simulink model "FO_CTDNN_P_Bia_Para_3_trigger_V1"  (R2021b)
settings: Solver=ode5  StartTime=0.0  StopTime=40  FixedStep=0.005  RelTol=1e-3
(part 1 of 2)
settings Model: Creator=a1752760  LastModifiedBy=a1752760
settings SolverCC: AlgebraicLoopSolver=TrustRegion
settings DebuggingCC: SFMachineParentedDataDiag=warning

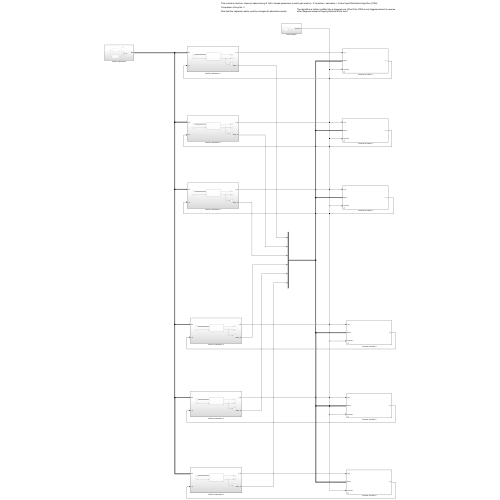
[thumbnail: Simulink's stored preview of the top-level diagram]
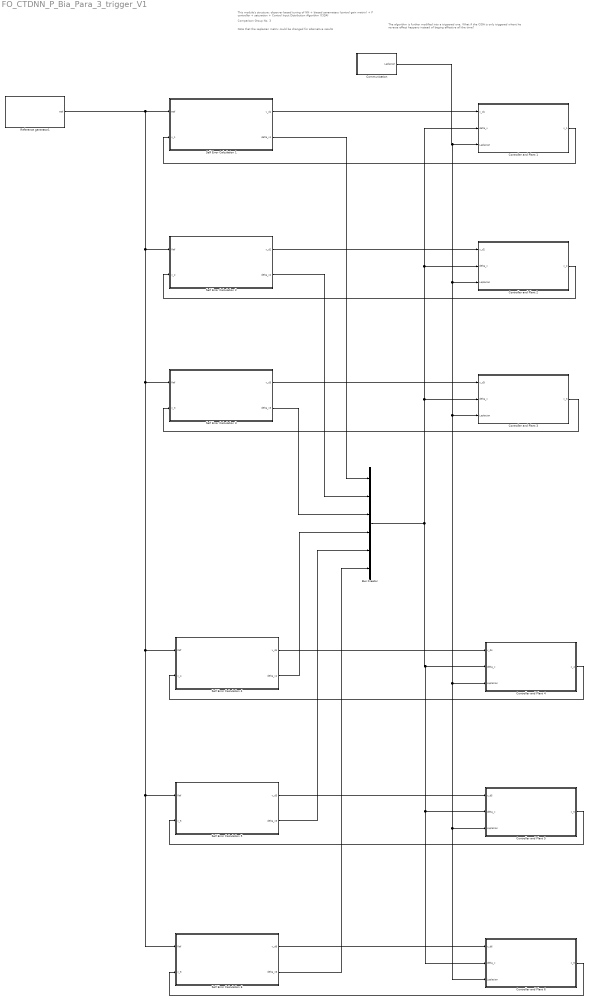
== system FO_CTDNN_P_Bia_Para_3_trigger_V1 ==
  note: The algorithm is further modified into a triggered one. What if the CIDA is only triggered whent he reverse
      | effect happens instead of beging effective all the time?
  note: Comparison Group No. 3
  note: This module's structure: observer based tuning of NN + biased parameters (control gain matrix) + P controller + saturation + Control Input Distribution Algorithm (CIDA)
  note: Note that the Laplacian matrix could be changed for alternative results
  Bus Creator : BusCreator  Inputs=6
  Communication : Subsystem
  Controller and Plant 1 : Subsystem  mask{InitialCondition=[-0.2;-0.7;-pi/4], UpperLimit=0.25, LowerLimit=-0.25}
      mask prompts: InitialCondition "Simulink:blkprm_prompts:IntegratorInitCond"; UpperLimit "Simulink:blkprm_prompts:SaturateUpLim"; LowerLimit "Simulink:blkprm_prompts:SaturateLowLim"
      mask TypeOptions InitialCondition: x_int/InitialCondition
      mask TypeOptions UpperLimit: Saturation/UpperLimit
      mask TypeOptions LowerLimit: Saturation/LowerLimit
      mask DialogControl InitialCondition Prompt: Initial condition:
      mask DialogControl UpperLimit Prompt: Upper limit:
      mask DialogControl LowerLimit Prompt: Lower limit:
  Controller and Plant 2 : Subsystem  mask{InitialCondition=[1.6;3.6;-pi/5], UpperLimit=0.25, LowerLimit=-0.25}
      mask prompts: InitialCondition "Simulink:blkprm_prompts:IntegratorInitCond"; UpperLimit "Simulink:blkprm_prompts:SaturateUpLim"; LowerLimit "Simulink:blkprm_prompts:SaturateLowLim"
      mask TypeOptions InitialCondition: x_int/InitialCondition
      mask TypeOptions UpperLimit: Saturation/UpperLimit
      mask TypeOptions LowerLimit: Saturation/LowerLimit
      mask DialogControl InitialCondition Prompt: Initial condition:
      mask DialogControl UpperLimit Prompt: Upper limit:
      mask DialogControl LowerLimit Prompt: Lower limit:
  Controller and Plant 3 : Subsystem  mask{InitialCondition=[-4;-2.4;pi/3], UpperLimit=0.25, LowerLimit=-0.25}
      mask prompts: InitialCondition "Simulink:blkprm_prompts:IntegratorInitCond"; UpperLimit "Simulink:blkprm_prompts:SaturateUpLim"; LowerLimit "Simulink:blkprm_prompts:SaturateLowLim"
      mask TypeOptions InitialCondition: x_int/InitialCondition
      mask TypeOptions UpperLimit: Saturation/UpperLimit
      mask TypeOptions LowerLimit: Saturation/LowerLimit
      mask DialogControl InitialCondition Prompt: Initial condition:
      mask DialogControl UpperLimit Prompt: Upper limit:
      mask DialogControl LowerLimit Prompt: Lower limit:
  Controller and Plant 4 : Subsystem  mask{InitialCondition=[-1.9;-1.1;pi/4], UpperLimit=0.25, LowerLimit=-0.25}
      mask prompts: InitialCondition "Simulink:blkprm_prompts:IntegratorInitCond"; UpperLimit "Simulink:blkprm_prompts:SaturateUpLim"; LowerLimit "Simulink:blkprm_prompts:SaturateLowLim"
      mask TypeOptions InitialCondition: x_int/InitialCondition
      mask TypeOptions UpperLimit: Saturation/UpperLimit
      mask TypeOptions LowerLimit: Saturation/LowerLimit
      mask DialogControl InitialCondition Prompt: Initial condition:
      mask DialogControl UpperLimit Prompt: Upper limit:
      mask DialogControl LowerLimit Prompt: Lower limit:
  Controller and Plant 5 : Subsystem  mask{InitialCondition=[-1.6;-4.6;-pi/3], UpperLimit=0.25, LowerLimit=-0.25}
      mask prompts: InitialCondition "Simulink:blkprm_prompts:IntegratorInitCond"; UpperLimit "Simulink:blkprm_prompts:SaturateUpLim"; LowerLimit "Simulink:blkprm_prompts:SaturateLowLim"
      mask TypeOptions InitialCondition: x_int/InitialCondition
      mask TypeOptions UpperLimit: Saturation/UpperLimit
      mask TypeOptions LowerLimit: Saturation/LowerLimit
      mask DialogControl InitialCondition Prompt: Initial condition:
      mask DialogControl UpperLimit Prompt: Upper limit:
      mask DialogControl LowerLimit Prompt: Lower limit:
  Controller and Plant 6 : Subsystem  mask{InitialCondition=[3.6;-1.5;-pi/6], UpperLimit=0.25, LowerLimit=-0.25}
      mask prompts: InitialCondition "Simulink:blkprm_prompts:IntegratorInitCond"; UpperLimit "Simulink:blkprm_prompts:SaturateUpLim"; LowerLimit "Simulink:blkprm_prompts:SaturateLowLim"
      mask TypeOptions InitialCondition: x_int/InitialCondition
      mask TypeOptions UpperLimit: Saturation/UpperLimit
      mask TypeOptions LowerLimit: Saturation/LowerLimit
      mask DialogControl InitialCondition Prompt: Initial condition:
      mask DialogControl UpperLimit Prompt: Upper limit:
      mask DialogControl LowerLimit Prompt: Lower limit:
  Reference generator1 : Subsystem
  Self Error Calculation 1 : Subsystem
  Self Error Calculation 2 : Subsystem
  Self Error Calculation 3 : Subsystem
  Self Error Calculation 4 : Subsystem
  Self Error Calculation 5 : Subsystem
  Self Error Calculation 6 : Subsystem
  wires:
  Reference generator1/1(Ref) -> Self Error Calculation 6/1(Ref), Self Error Calculation 5/1(Ref), Self Error Calculation 4/1(Ref), Self Error Calculation 3/1(Ref), Self Error Calculation 2/1(Ref), Self Error Calculation 1/1(Ref)
  Self Error Calculation 1/1(v_d1) -> Controller and Plant 1/1(v_d1)
  Controller and Plant 1/1(x_1) -> Self Error Calculation 1/2(x_1)
  Controller and Plant 2/1(x_2) -> Self Error Calculation 2/2(x_2)
  Self Error Calculation 2/1(v_d2) -> Controller and Plant 2/1(v_d2)
  Controller and Plant 3/1(x_3) -> Self Error Calculation 3/2(x_3)
  Self Error Calculation 3/1(v_d3) -> Controller and Plant 3/1(v_d3)
  Controller and Plant 4/1(x_4) -> Self Error Calculation 4/2(x_4)
  Self Error Calculation 4/1(v_d4) -> Controller and Plant 4/1(v_d4)
  Controller and Plant 5/1(x_5) -> Self Error Calculation 5/2(x_5)
  Self Error Calculation 5/1(v_d5) -> Controller and Plant 5/1(v_d5)
  Controller and Plant 6/1(x_6) -> Self Error Calculation 6/2(x_6)
  Self Error Calculation 6/1(v_d6) -> Controller and Plant 6/1(v_d6)
  Self Error Calculation 1/2(delta_x1) -> Bus Creator/1
  Self Error Calculation 2/2(delta_x2) -> Bus Creator/2
  Self Error Calculation 3/2(delta_x3) -> Bus Creator/3
  Self Error Calculation 4/2(delta_x4) -> Bus Creator/4
  Self Error Calculation 5/2(delta_x5) -> Bus Creator/5
  Self Error Calculation 6/2(delta_x6) -> Bus Creator/6
  Bus Creator/1 -> Controller and Plant 4/2(delta_x), Controller and Plant 6/2(delta_x), Controller and Plant 5/2(delta_x), Controller and Plant 3/2(delta_x), Controller and Plant 2/2(delta_x), Controller and Plant 1/2(delta_x)
  Communication/1(Laplacian) -> Controller and Plant 6/3(Laplacian), Controller and Plant 5/3(Laplacian), Controller and Plant 4/3(Laplacian), Controller and Plant 3/3(Laplacian), Controller and Plant 2/3(Laplacian), Controller and Plant 1/3(Laplacian)

== system FO_CTDNN_P_Bia_Para_3_trigger_V1/Communication ==
  Add : Sum
  Communication Topology : Constant  Value=[2,0,-1,-1,0,0;-1,1,0,0,0,0;0,-1,2,-1,0,0;-1,0,0,3,-1,-1;0,0,0,-1,1,0;-1,0,0,0,0,1]  VectorParams1D=off
  Constant : Constant  Value=2  VectorParams1D=off
  Product : Product
  Reference Feeding : Constant  Value=[1,0,0,0,0,0;0,1,0,0,0,0;0,0,1,0,0,0;0,0,0,1,0,0;0,0,0,0,1,0;0,0,0,0,0,1]  VectorParams1D=off
  Laplacian : Outport  VectorParamsAs1DForOutWhenUnconnected=off
  wires:
  Constant/1 -> Product/2
  Reference Feeding/1 -> Product/1
  Communication Topology/1 -> Add/1
  Product/1 -> Add/2
  Add/1 -> Laplacian/1

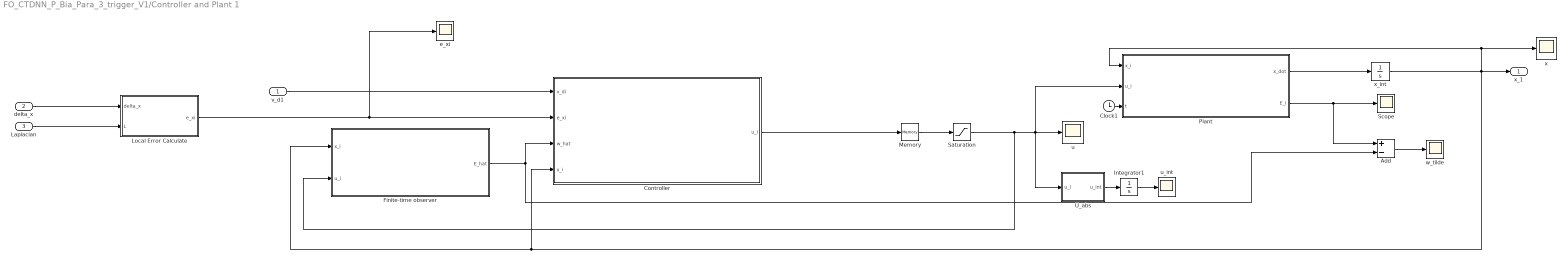
== system FO_CTDNN_P_Bia_Para_3_trigger_V1/Controller and Plant 1 ==
  v_d1 : Inport
  delta_x : Inport  Port=2
  Laplacian : Inport  Port=3
  Add : Sum  Inputs=+-
  Clock1 : Clock
  Controller : Subsystem
  Finite-time observer : Subsystem  mask{InitialCondition=[0;-0.3;-pi/5]}
      mask prompts: InitialCondition "Simulink:blkprm_prompts:IntegratorInitCond"
      mask TypeOptions InitialCondition: Integrator/InitialCondition
      mask DialogControl InitialCondition Prompt: Initial condition:
  Integrator1 : Integrator
  Local Error Calculate : MATLAB Function  TreatAsAtomicUnit=on
  Memory : Memory  InitialCondition=[0;0;0]
  Plant : MATLAB Function  TreatAsAtomicUnit=on
  Saturation : Saturate  UpperLimit=UpperLimit  LowerLimit=LowerLimit
  Scope : Scope
  U_abs : MATLAB Function  TreatAsAtomicUnit=on
  e_xi : Scope
  u : Scope
  u_int : Scope
  w_tilde : Scope
  x : Scope
  x_int : Integrator  InitialCondition=InitialCondition
  x_1 : Outport
  wires:
  Add/1 -> w_tilde/1
  Plant/2(E_i) -> Scope/1, Add/1
  Finite-time observer/1(E_hat) -> Controller/3(w_hat), Add/2
  Clock1/1 -> Plant/3(t)
  Plant/1(x_dot) -> x_int/1
  Memory/1 -> Saturation/1
  x_int/1 -> x_1/1, Plant/1(x_i), x/1, Controller/4(x_i), Finite-time observer/1(x_i)
  v_d1/1 -> Controller/1(v_di)
  Controller/1(u_i) -> Memory/1
  Local Error Calculate/1(e_xi) -> Controller/2(e_xi), e_xi/1
  delta_x/1 -> Local Error Calculate/1(delta_x)
  Laplacian/1 -> Local Error Calculate/2(L)
  Saturation/1 -> Finite-time observer/2(u_i), U_abs/1(u_i), Plant/2(u_i), u/1
  Integrator1/1 -> u_int/1
  U_abs/1(u_int) -> Integrator1/1

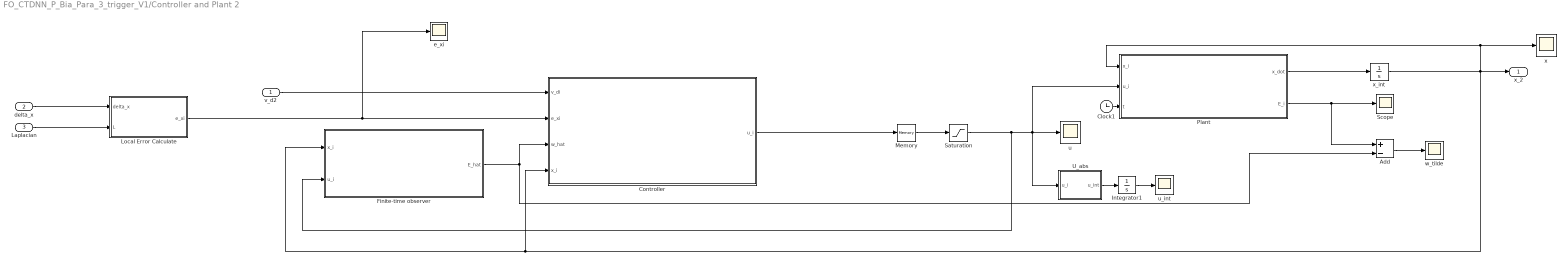
== system FO_CTDNN_P_Bia_Para_3_trigger_V1/Controller and Plant 2 ==
  v_d2 : Inport
  delta_x : Inport  Port=2
  Laplacian : Inport  Port=3
  Add : Sum  Inputs=+-
  Clock1 : Clock
  Controller : Subsystem
  Finite-time observer : Subsystem  mask{InitialCondition=[1.4;3.3;-pi/6]}
      mask prompts: InitialCondition "Simulink:blkprm_prompts:IntegratorInitCond"
      mask TypeOptions InitialCondition: Integrator/InitialCondition
      mask DialogControl InitialCondition Prompt: Initial condition:
  Integrator1 : Integrator
  Local Error Calculate : MATLAB Function  TreatAsAtomicUnit=on
  Memory : Memory  InitialCondition=[0;0;0]
  Plant : MATLAB Function  TreatAsAtomicUnit=on
  Saturation : Saturate  UpperLimit=UpperLimit  LowerLimit=LowerLimit
  Scope : Scope
  U_abs : MATLAB Function  TreatAsAtomicUnit=on
  e_xi : Scope
  u : Scope
  u_int : Scope
  w_tilde : Scope
  x : Scope
  x_int : Integrator  InitialCondition=InitialCondition
  x_2 : Outport
  wires:
  Add/1 -> w_tilde/1
  Plant/2(E_i) -> Scope/1, Add/1
  Finite-time observer/1(E_hat) -> Controller/3(w_hat), Add/2
  Clock1/1 -> Plant/3(t)
  Plant/1(x_dot) -> x_int/1
  Memory/1 -> Saturation/1
  x_int/1 -> x_2/1, Plant/1(x_i), x/1, Controller/4(x_i), Finite-time observer/1(x_i)
  v_d2/1 -> Controller/1(v_di)
  Controller/1(u_i) -> Memory/1
  Local Error Calculate/1(e_xi) -> Controller/2(e_xi), e_xi/1
  delta_x/1 -> Local Error Calculate/1(delta_x)
  Laplacian/1 -> Local Error Calculate/2(L)
  Integrator1/1 -> u_int/1
  Saturation/1 -> Finite-time observer/2(u_i), U_abs/1(u_i), Plant/2(u_i), u/1
  U_abs/1(u_int) -> Integrator1/1

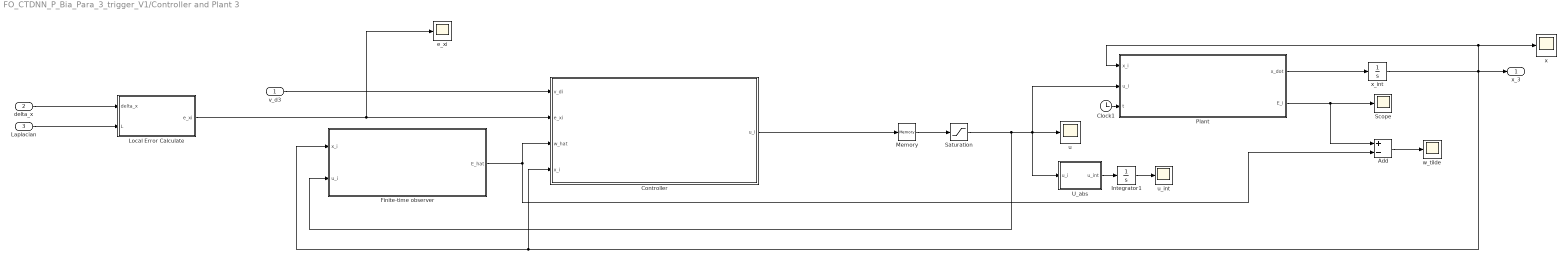
== system FO_CTDNN_P_Bia_Para_3_trigger_V1/Controller and Plant 3 ==
  v_d3 : Inport
  delta_x : Inport  Port=2
  Laplacian : Inport  Port=3
  Add : Sum  Inputs=+-
  Clock1 : Clock
  Controller : Subsystem
  Finite-time observer : Subsystem  mask{InitialCondition=[-3.7;-2.1;pi/4]}
      mask prompts: InitialCondition "Simulink:blkprm_prompts:IntegratorInitCond"
      mask TypeOptions InitialCondition: Integrator/InitialCondition
      mask DialogControl InitialCondition Prompt: Initial condition:
  Integrator1 : Integrator
  Local Error Calculate : MATLAB Function  TreatAsAtomicUnit=on
  Memory : Memory  InitialCondition=[0;0;0]
  Plant : MATLAB Function  TreatAsAtomicUnit=on
  Saturation : Saturate  UpperLimit=UpperLimit  LowerLimit=LowerLimit
  Scope : Scope
  U_abs : MATLAB Function  TreatAsAtomicUnit=on
  e_xi : Scope
  u : Scope
  u_int : Scope
  w_tilde : Scope
  x : Scope
  x_int : Integrator  InitialCondition=InitialCondition
  x_3 : Outport
  wires:
  Add/1 -> w_tilde/1
  Plant/2(E_i) -> Scope/1, Add/1
  Finite-time observer/1(E_hat) -> Controller/3(w_hat), Add/2
  Clock1/1 -> Plant/3(t)
  Plant/1(x_dot) -> x_int/1
  Memory/1 -> Saturation/1
  x_int/1 -> x_3/1, Plant/1(x_i), x/1, Controller/4(x_i), Finite-time observer/1(x_i)
  v_d3/1 -> Controller/1(v_di)
  Controller/1(u_i) -> Memory/1
  Local Error Calculate/1(e_xi) -> Controller/2(e_xi), e_xi/1
  delta_x/1 -> Local Error Calculate/1(delta_x)
  Laplacian/1 -> Local Error Calculate/2(L)
  Integrator1/1 -> u_int/1
  Saturation/1 -> Finite-time observer/2(u_i), U_abs/1(u_i), Plant/2(u_i), u/1
  U_abs/1(u_int) -> Integrator1/1

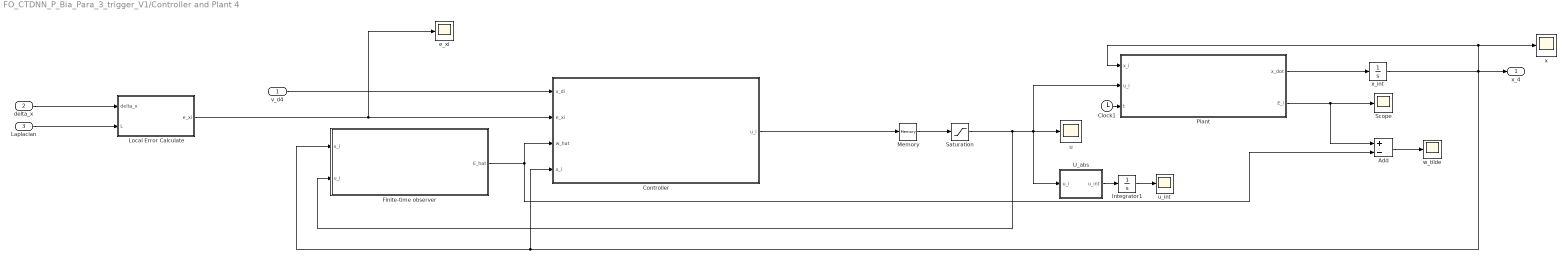
== system FO_CTDNN_P_Bia_Para_3_trigger_V1/Controller and Plant 4 ==
  v_d4 : Inport
  delta_x : Inport  Port=2
  Laplacian : Inport  Port=3
  Add : Sum  Inputs=+-
  Clock1 : Clock
  Controller : Subsystem
  Finite-time observer : Subsystem  mask{InitialCondition=[-1.6;-0.8;pi/6]}
      mask prompts: InitialCondition "Simulink:blkprm_prompts:IntegratorInitCond"
      mask TypeOptions InitialCondition: Integrator/InitialCondition
      mask DialogControl InitialCondition Prompt: Initial condition:
  Integrator1 : Integrator
  Local Error Calculate : MATLAB Function  TreatAsAtomicUnit=on
  Memory : Memory  InitialCondition=[0;0;0]
  Plant : MATLAB Function  TreatAsAtomicUnit=on
  Saturation : Saturate  UpperLimit=UpperLimit  LowerLimit=LowerLimit
  Scope : Scope
  U_abs : MATLAB Function  TreatAsAtomicUnit=on
  e_xi : Scope
  u : Scope
  u_int : Scope
  w_tilde : Scope
  x : Scope
  x_int : Integrator  InitialCondition=InitialCondition
  x_4 : Outport
  wires:
  Add/1 -> w_tilde/1
  Plant/2(E_i) -> Scope/1, Add/1
  Finite-time observer/1(E_hat) -> Controller/3(w_hat), Add/2
  Clock1/1 -> Plant/3(t)
  Plant/1(x_dot) -> x_int/1
  Memory/1 -> Saturation/1
  x_int/1 -> x_4/1, Plant/1(x_i), x/1, Controller/4(x_i), Finite-time observer/1(x_i)
  v_d4/1 -> Controller/1(v_di)
  Controller/1(u_i) -> Memory/1
  Local Error Calculate/1(e_xi) -> Controller/2(e_xi), e_xi/1
  delta_x/1 -> Local Error Calculate/1(delta_x)
  Laplacian/1 -> Local Error Calculate/2(L)
  U_abs/1(u_int) -> Integrator1/1
  Integrator1/1 -> u_int/1
  Saturation/1 -> Finite-time observer/2(u_i), U_abs/1(u_i), Plant/2(u_i), u/1

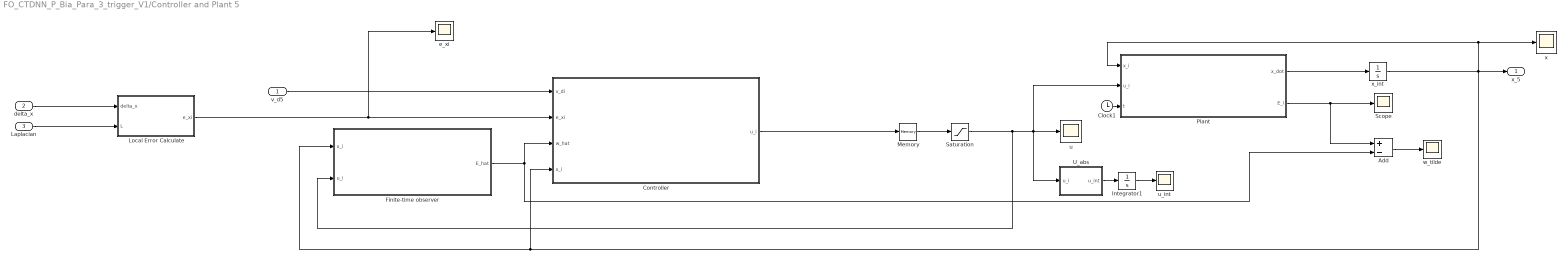
== system FO_CTDNN_P_Bia_Para_3_trigger_V1/Controller and Plant 5 ==
  v_d5 : Inport
  delta_x : Inport  Port=2
  Laplacian : Inport  Port=3
  Add : Sum  Inputs=+-
  Clock1 : Clock
  Controller : Subsystem
  Finite-time observer : Subsystem  mask{InitialCondition=[-1.1;-4.1;-pi/4]}
      mask prompts: InitialCondition "Simulink:blkprm_prompts:IntegratorInitCond"
      mask TypeOptions InitialCondition: Integrator/InitialCondition
      mask DialogControl InitialCondition Prompt: Initial condition:
  Integrator1 : Integrator
  Local Error Calculate : MATLAB Function  TreatAsAtomicUnit=on
  Memory : Memory  InitialCondition=[0;0;0]
  Plant : MATLAB Function  TreatAsAtomicUnit=on
  Saturation : Saturate  UpperLimit=UpperLimit  LowerLimit=LowerLimit
  Scope : Scope
  U_abs : MATLAB Function  TreatAsAtomicUnit=on
  e_xi : Scope
  u : Scope
  u_int : Scope
  w_tilde : Scope
  x : Scope
  x_int : Integrator  InitialCondition=InitialCondition
  x_5 : Outport
  wires:
  Add/1 -> w_tilde/1
  Plant/2(E_i) -> Scope/1, Add/1
  Finite-time observer/1(E_hat) -> Controller/3(w_hat), Add/2
  Clock1/1 -> Plant/3(t)
  Plant/1(x_dot) -> x_int/1
  Memory/1 -> Saturation/1
  x_int/1 -> x_5/1, Plant/1(x_i), x/1, Controller/4(x_i), Finite-time observer/1(x_i)
  v_d5/1 -> Controller/1(v_di)
  Controller/1(u_i) -> Memory/1
  Local Error Calculate/1(e_xi) -> Controller/2(e_xi), e_xi/1
  delta_x/1 -> Local Error Calculate/1(delta_x)
  Laplacian/1 -> Local Error Calculate/2(L)
  U_abs/1(u_int) -> Integrator1/1
  Integrator1/1 -> u_int/1
  Saturation/1 -> Finite-time observer/2(u_i), U_abs/1(u_i), Plant/2(u_i), u/1

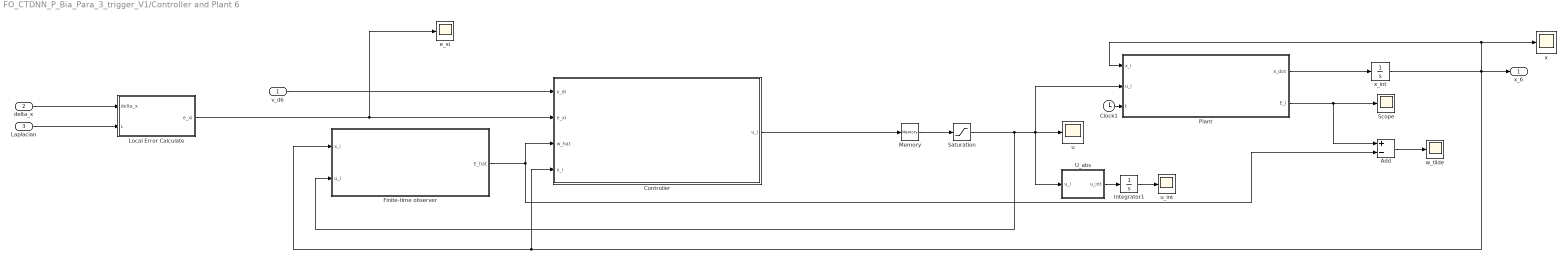
== system FO_CTDNN_P_Bia_Para_3_trigger_V1/Controller and Plant 6 ==
  v_d6 : Inport
  delta_x : Inport  Port=2
  Laplacian : Inport  Port=3
  Add : Sum  Inputs=+-
  Clock1 : Clock
  Controller : Subsystem
  Finite-time observer : Subsystem  mask{InitialCondition=[3.9;-1.9;-pi/5]}
      mask prompts: InitialCondition "Simulink:blkprm_prompts:IntegratorInitCond"
      mask TypeOptions InitialCondition: Integrator/InitialCondition
      mask DialogControl InitialCondition Prompt: Initial condition:
  Integrator1 : Integrator
  Local Error Calculate : MATLAB Function  TreatAsAtomicUnit=on
  Memory : Memory  InitialCondition=[0;0;0]
  Plant : MATLAB Function  TreatAsAtomicUnit=on
  Saturation : Saturate  UpperLimit=UpperLimit  LowerLimit=LowerLimit
  Scope : Scope
  U_abs : MATLAB Function  TreatAsAtomicUnit=on
  e_xi : Scope
  u : Scope
  u_int : Scope
  w_tilde : Scope
  x : Scope
  x_int : Integrator  InitialCondition=InitialCondition
  x_6 : Outport
  wires:
  Add/1 -> w_tilde/1
  Plant/2(E_i) -> Scope/1, Add/1
  Finite-time observer/1(E_hat) -> Controller/3(w_hat), Add/2
  Clock1/1 -> Plant/3(t)
  Plant/1(x_dot) -> x_int/1
  Memory/1 -> Saturation/1
  x_int/1 -> x_6/1, Plant/1(x_i), x/1, Controller/4(x_i), Finite-time observer/1(x_i)
  v_d6/1 -> Controller/1(v_di)
  Controller/1(u_i) -> Memory/1
  Local Error Calculate/1(e_xi) -> Controller/2(e_xi), e_xi/1
  delta_x/1 -> Local Error Calculate/1(delta_x)
  Laplacian/1 -> Local Error Calculate/2(L)
  U_abs/1(u_int) -> Integrator1/1
  Integrator1/1 -> u_int/1
  Saturation/1 -> Finite-time observer/2(u_i), U_abs/1(u_i), Plant/2(u_i), u/1

== system FO_CTDNN_P_Bia_Para_3_trigger_V1/Reference generator1 ==
  Bus Creator : BusCreator  Inputs=2
  Clock : Clock
  Scope : Scope
  reference : MATLAB Function  TreatAsAtomicUnit=on
  reference1 : MATLAB Function  TreatAsAtomicUnit=on
  Ref : Outport
  wires:
  Clock/1 -> reference1/1(t), reference/1(t)
  reference/1(xd) -> Scope/1, Bus Creator/1
  reference1/1(vd) -> Bus Creator/2
  Bus Creator/1 -> Ref/1

== system FO_CTDNN_P_Bia_Para_3_trigger_V1/Self Error Calculation 1 ==
  Ref : Inport
  x_1 : Inport  Port=2
  Scope : Scope
  error_calculation : MATLAB Function  TreatAsAtomicUnit=on
  v_d1 : Outport
  delta_x1 : Outport  Port=2
  wires:
  Ref/1 -> error_calculation/1(ref)
  x_1/1 -> error_calculation/2(x_i)
  error_calculation/1(v_di) -> v_d1/1
  error_calculation/2(delta_x1) -> Scope/1, delta_x1/1

== system FO_CTDNN_P_Bia_Para_3_trigger_V1/Self Error Calculation 2 ==
  Ref : Inport
  x_2 : Inport  Port=2
  Scope : Scope
  error_calculation : MATLAB Function  TreatAsAtomicUnit=on
  v_d2 : Outport
  delta_x2 : Outport  Port=2
  wires:
  Ref/1 -> error_calculation/1(ref)
  x_2/1 -> error_calculation/2(x_i)
  error_calculation/1(v_di) -> v_d2/1
  error_calculation/2(delta_x2) -> Scope/1, delta_x2/1

== system FO_CTDNN_P_Bia_Para_3_trigger_V1/Self Error Calculation 3 ==
  Ref : Inport
  x_3 : Inport  Port=2
  Scope : Scope
  error_calculation : MATLAB Function  TreatAsAtomicUnit=on
  v_d3 : Outport
  delta_x3 : Outport  Port=2
  wires:
  Ref/1 -> error_calculation/1(ref)
  x_3/1 -> error_calculation/2(x_i)
  error_calculation/1(v_di) -> v_d3/1
  error_calculation/2(delta_x3) -> Scope/1, delta_x3/1

== system FO_CTDNN_P_Bia_Para_3_trigger_V1/Self Error Calculation 4 ==
  Ref : Inport
  x_4 : Inport  Port=2
  Scope : Scope
  error_calculation : MATLAB Function  TreatAsAtomicUnit=on
  v_d4 : Outport
  delta_x4 : Outport  Port=2
  wires:
  Ref/1 -> error_calculation/1(ref)
  x_4/1 -> error_calculation/2(x_i)
  error_calculation/1(v_di) -> v_d4/1
  error_calculation/2(delta_x4) -> Scope/1, delta_x4/1

== system FO_CTDNN_P_Bia_Para_3_trigger_V1/Self Error Calculation 5 ==
  Ref : Inport
  x_5 : Inport  Port=2
  Scope : Scope
  error_calculation : MATLAB Function  TreatAsAtomicUnit=on
  v_d5 : Outport
  delta_x5 : Outport  Port=2
  wires:
  Ref/1 -> error_calculation/1(ref)
  x_5/1 -> error_calculation/2(x_i)
  error_calculation/1(v_di) -> v_d5/1
  error_calculation/2(delta_x5) -> Scope/1, delta_x5/1

== system FO_CTDNN_P_Bia_Para_3_trigger_V1/Self Error Calculation 6 ==
  Ref : Inport
  x_6 : Inport  Port=2
  Scope : Scope
  error_calculation : MATLAB Function  TreatAsAtomicUnit=on
  v_d6 : Outport
  delta_x6 : Outport  Port=2
  wires:
  Ref/1 -> error_calculation/1(ref)
  x_6/1 -> error_calculation/2(x_i)
  error_calculation/1(v_di) -> v_d6/1
  error_calculation/2(delta_x6) -> Scope/1, delta_x6/1

== system FO_CTDNN_P_Bia_Para_3_trigger_V1/Controller and Plant 1/Controller ==
  v_di : Inport
  e_xi : Inport  Port=2
  w_hat : Inport  Port=3
  x_i : Inport  Port=4
  Add : Sum
  Control gain matrix : MATLAB Function  TreatAsAtomicUnit=on
  Scope{,1..3} (4 alike) : Scope
  Smooth Projection : MATLAB Function  TreatAsAtomicUnit=on
  controller : MATLAB Function  TreatAsAtomicUnit=on
  u_d,i : MATLAB Function  TreatAsAtomicUnit=on
  u_e,i : MATLAB Function  TreatAsAtomicUnit=on
  u_t,i : MATLAB Function  TreatAsAtomicUnit=on
  xi_i : Scope
  u_i : Outport
  wires:
  x_i/1 -> Control gain matrix/1(x_i)
  Control gain matrix/2(g_inverse) -> u_e,i/1(g_inverse), u_d,i/1(g_inverse), u_t,i/1(g_inverse)
  v_di/1 -> u_t,i/2(v_di)
  w_hat/1 -> Scope3/1, u_d,i/2(w_hat)
  e_xi/1 -> u_e,i/2(e_xi)
  u_e,i/1(u_ei) -> controller/3(u_ei), Scope/1
  controller/1(u_i) -> u_i/1
  controller/2(xi_min) -> xi_i/1
  u_t,i/1(u_ti) -> Add/1
  u_d,i/1(u_di) -> Add/2
  Add/1 -> Scope1/1, Smooth Projection/1("u_mi ")
  Smooth Projection/1(u_mi) -> controller/2(u_mi), Scope2/1
  Control gain matrix/1(g_i_hat) -> controller/1(g_i_hat)

== system FO_CTDNN_P_Bia_Para_3_trigger_V1/Controller and Plant 1/Finite-time observer ==
  x_i : Inport
  u_i : Inport  Port=2
  Integrator : Integrator  InitialCondition=InitialCondition
  Multi-layer neural network : Subsystem
  Observer : MATLAB Function  TreatAsAtomicUnit=on
  x_i_tilde : Scope
  E_hat : Outport
  wires:
  x_i/1 -> Observer/2(x_i), Multi-layer neural network/2(x_i)
  u_i/1 -> Observer/3(u_i), Multi-layer neural network/3(u_i)
  Multi-layer neural network/1(E_hat) -> E_hat/1, Observer/4(E_hat)
  Observer/1(x_hat_dot) -> Integrator/1
  Integrator/1 -> Observer/1(x_i_hat)
  Observer/2(x_i_tilde) -> x_i_tilde/1, Multi-layer neural network/1(x_i_tilde)

== system FO_CTDNN_P_Bia_Para_3_trigger_V1/Controller and Plant 2/Controller ==
  v_di : Inport
  e_xi : Inport  Port=2
  w_hat : Inport  Port=3
  x_i : Inport  Port=4
  Add : Sum
  Control gain matrix : MATLAB Function  TreatAsAtomicUnit=on
  Scope{,1..3} (4 alike) : Scope
  Smooth Projection : MATLAB Function  TreatAsAtomicUnit=on
  controller : MATLAB Function  TreatAsAtomicUnit=on
  u_d,i : MATLAB Function  TreatAsAtomicUnit=on
  u_e,i : MATLAB Function  TreatAsAtomicUnit=on
  u_t,i : MATLAB Function  TreatAsAtomicUnit=on
  xi_i : Scope
  u_i : Outport
  wires:
  x_i/1 -> Control gain matrix/1(x_i)
  Control gain matrix/2(g_inverse) -> u_e,i/1(g_inverse), u_d,i/1(g_inverse), u_t,i/1(g_inverse)
  v_di/1 -> u_t,i/2(v_di)
  w_hat/1 -> Scope3/1, u_d,i/2(w_hat)
  e_xi/1 -> u_e,i/2(e_xi)
  u_e,i/1(u_ei) -> controller/3(u_ei), Scope/1
  controller/1(u_i) -> u_i/1
  controller/2(xi_min) -> xi_i/1
  u_t,i/1(u_ti) -> Add/1
  u_d,i/1(u_di) -> Add/2
  Add/1 -> Scope1/1, Smooth Projection/1("u_mi ")
  Smooth Projection/1(u_mi) -> controller/2(u_mi), Scope2/1
  Control gain matrix/1(g_i_hat) -> controller/1(g_i_hat)

== system FO_CTDNN_P_Bia_Para_3_trigger_V1/Controller and Plant 2/Finite-time observer ==
  x_i : Inport
  u_i : Inport  Port=2
  Integrator : Integrator  InitialCondition=InitialCondition
  Multi-layer neural network : Subsystem
  Observer : MATLAB Function  TreatAsAtomicUnit=on
  x_i_tilde : Scope
  E_hat : Outport
  wires:
  x_i/1 -> Observer/2(x_i), Multi-layer neural network/2(x_i)
  u_i/1 -> Observer/3(u_i), Multi-layer neural network/3(u_i)
  Multi-layer neural network/1(E_hat) -> E_hat/1, Observer/4(E_hat)
  Observer/1(x_hat_dot) -> Integrator/1
  Integrator/1 -> Observer/1(x_i_hat)
  Observer/2(x_i_tilde) -> x_i_tilde/1, Multi-layer neural network/1(x_i_tilde)

== system FO_CTDNN_P_Bia_Para_3_trigger_V1/Controller and Plant 3/Controller ==
  v_di : Inport
  e_xi : Inport  Port=2
  w_hat : Inport  Port=3
  x_i : Inport  Port=4
  Add : Sum
  Control gain matrix : MATLAB Function  TreatAsAtomicUnit=on
  Scope{,1..3} (4 alike) : Scope
  Smooth Projection : MATLAB Function  TreatAsAtomicUnit=on
  controller : MATLAB Function  TreatAsAtomicUnit=on
  u_d,i : MATLAB Function  TreatAsAtomicUnit=on
  u_e,i : MATLAB Function  TreatAsAtomicUnit=on
  u_t,i : MATLAB Function  TreatAsAtomicUnit=on
  xi_i : Scope
  u_i : Outport
  wires:
  x_i/1 -> Control gain matrix/1(x_i)
  Control gain matrix/2(g_inverse) -> u_e,i/1(g_inverse), u_d,i/1(g_inverse), u_t,i/1(g_inverse)
  v_di/1 -> u_t,i/2(v_di)
  w_hat/1 -> Scope3/1, u_d,i/2(w_hat)
  e_xi/1 -> u_e,i/2(e_xi)
  u_e,i/1(u_ei) -> controller/3(u_ei), Scope/1
  controller/1(u_i) -> u_i/1
  controller/2(xi_min) -> xi_i/1
  u_t,i/1(u_ti) -> Add/1
  u_d,i/1(u_di) -> Add/2
  Add/1 -> Scope1/1, Smooth Projection/1("u_mi ")
  Smooth Projection/1(u_mi) -> controller/2(u_mi), Scope2/1
  Control gain matrix/1(g_i_hat) -> controller/1(g_i_hat)

== system FO_CTDNN_P_Bia_Para_3_trigger_V1/Controller and Plant 3/Finite-time observer ==
  x_i : Inport
  u_i : Inport  Port=2
  Integrator : Integrator  InitialCondition=InitialCondition
  Multi-layer neural network : Subsystem
  Observer : MATLAB Function  TreatAsAtomicUnit=on
  x_i_tilde : Scope
  E_hat : Outport
  wires:
  x_i/1 -> Observer/2(x_i), Multi-layer neural network/2(x_i)
  u_i/1 -> Observer/3(u_i), Multi-layer neural network/3(u_i)
  Multi-layer neural network/1(E_hat) -> E_hat/1, Observer/4(E_hat)
  Observer/1(x_hat_dot) -> Integrator/1
  Integrator/1 -> Observer/1(x_i_hat)
  Observer/2(x_i_tilde) -> x_i_tilde/1, Multi-layer neural network/1(x_i_tilde)

== system FO_CTDNN_P_Bia_Para_3_trigger_V1/Controller and Plant 4/Controller ==
  v_di : Inport
  e_xi : Inport  Port=2
  w_hat : Inport  Port=3
  x_i : Inport  Port=4
  Add : Sum
  Control gain matrix : MATLAB Function  TreatAsAtomicUnit=on
  Scope{,1..3} (4 alike) : Scope
  Smooth Projection : MATLAB Function  TreatAsAtomicUnit=on
  controller : MATLAB Function  TreatAsAtomicUnit=on
  u_d,i : MATLAB Function  TreatAsAtomicUnit=on
  u_e,i : MATLAB Function  TreatAsAtomicUnit=on
  u_t,i : MATLAB Function  TreatAsAtomicUnit=on
  xi_i : Scope
  u_i : Outport
  wires:
  x_i/1 -> Control gain matrix/1(x_i)
  Control gain matrix/2(g_inverse) -> u_e,i/1(g_inverse), u_d,i/1(g_inverse), u_t,i/1(g_inverse)
  v_di/1 -> u_t,i/2(v_di)
  w_hat/1 -> Scope3/1, u_d,i/2(w_hat)
  e_xi/1 -> u_e,i/2(e_xi)
  u_e,i/1(u_ei) -> controller/3(u_ei), Scope/1
  controller/1(u_i) -> u_i/1
  controller/2(xi_min) -> xi_i/1
  u_t,i/1(u_ti) -> Add/1
  u_d,i/1(u_di) -> Add/2
  Add/1 -> Scope1/1, Smooth Projection/1("u_mi ")
  Smooth Projection/1(u_mi) -> controller/2(u_mi), Scope2/1
  Control gain matrix/1(g_i_hat) -> controller/1(g_i_hat)

== system FO_CTDNN_P_Bia_Para_3_trigger_V1/Controller and Plant 4/Finite-time observer ==
  x_i : Inport
  u_i : Inport  Port=2
  Integrator : Integrator  InitialCondition=InitialCondition
  Multi-layer neural network : Subsystem
  Observer : MATLAB Function  TreatAsAtomicUnit=on
  x_i_tilde : Scope
  E_hat : Outport
  wires:
  x_i/1 -> Observer/2(x_i), Multi-layer neural network/2(x_i)
  u_i/1 -> Observer/3(u_i), Multi-layer neural network/3(u_i)
  Multi-layer neural network/1(E_hat) -> E_hat/1, Observer/4(E_hat)
  Observer/1(x_hat_dot) -> Integrator/1
  Integrator/1 -> Observer/1(x_i_hat)
  Observer/2(x_i_tilde) -> x_i_tilde/1, Multi-layer neural network/1(x_i_tilde)

== system FO_CTDNN_P_Bia_Para_3_trigger_V1/Controller and Plant 5/Controller ==
  v_di : Inport
  e_xi : Inport  Port=2
  w_hat : Inport  Port=3
  x_i : Inport  Port=4
  Add : Sum
  Control gain matrix : MATLAB Function  TreatAsAtomicUnit=on
  Scope{,1..3} (4 alike) : Scope
  Smooth Projection : MATLAB Function  TreatAsAtomicUnit=on
  controller : MATLAB Function  TreatAsAtomicUnit=on
  u_d,i : MATLAB Function  TreatAsAtomicUnit=on
  u_e,i : MATLAB Function  TreatAsAtomicUnit=on
  u_t,i : MATLAB Function  TreatAsAtomicUnit=on
  xi_i : Scope
  u_i : Outport
  wires:
  x_i/1 -> Control gain matrix/1(x_i)
  Control gain matrix/2(g_inverse) -> u_e,i/1(g_inverse), u_d,i/1(g_inverse), u_t,i/1(g_inverse)
  v_di/1 -> u_t,i/2(v_di)
  w_hat/1 -> Scope3/1, u_d,i/2(w_hat)
  e_xi/1 -> u_e,i/2(e_xi)
  u_e,i/1(u_ei) -> controller/3(u_ei), Scope/1
  controller/1(u_i) -> u_i/1
  controller/2(xi_min) -> xi_i/1
  u_t,i/1(u_ti) -> Add/1
  u_d,i/1(u_di) -> Add/2
  Add/1 -> Scope1/1, Smooth Projection/1("u_mi ")
  Smooth Projection/1(u_mi) -> controller/2(u_mi), Scope2/1
  Control gain matrix/1(g_i_hat) -> controller/1(g_i_hat)

== system FO_CTDNN_P_Bia_Para_3_trigger_V1/Controller and Plant 5/Finite-time observer ==
  x_i : Inport
  u_i : Inport  Port=2
  Integrator : Integrator  InitialCondition=InitialCondition
  Multi-layer neural network : Subsystem
  Observer : MATLAB Function  TreatAsAtomicUnit=on
  x_i_tilde : Scope
  E_hat : Outport
  wires:
  x_i/1 -> Observer/2(x_i), Multi-layer neural network/2(x_i)
  u_i/1 -> Observer/3(u_i), Multi-layer neural network/3(u_i)
  Multi-layer neural network/1(E_hat) -> E_hat/1, Observer/4(E_hat)
  Observer/1(x_hat_dot) -> Integrator/1
  Integrator/1 -> Observer/1(x_i_hat)
  Observer/2(x_i_tilde) -> x_i_tilde/1, Multi-layer neural network/1(x_i_tilde)

== system FO_CTDNN_P_Bia_Para_3_trigger_V1/Controller and Plant 6/Controller ==
  v_di : Inport
  e_xi : Inport  Port=2
  w_hat : Inport  Port=3
  x_i : Inport  Port=4
  Add : Sum
  Control gain matrix : MATLAB Function  TreatAsAtomicUnit=on
  Scope{,1..3} (4 alike) : Scope
  Smooth Projection : MATLAB Function  TreatAsAtomicUnit=on
  controller : MATLAB Function  TreatAsAtomicUnit=on
  u_d,i : MATLAB Function  TreatAsAtomicUnit=on
  u_e,i : MATLAB Function  TreatAsAtomicUnit=on
  u_t,i : MATLAB Function  TreatAsAtomicUnit=on
  xi_i : Scope
  u_i : Outport
  wires:
  x_i/1 -> Control gain matrix/1(x_i)
  Control gain matrix/2(g_inverse) -> u_e,i/1(g_inverse), u_d,i/1(g_inverse), u_t,i/1(g_inverse)
  v_di/1 -> u_t,i/2(v_di)
  w_hat/1 -> Scope3/1, u_d,i/2(w_hat)
  e_xi/1 -> u_e,i/2(e_xi)
  u_e,i/1(u_ei) -> controller/3(u_ei), Scope/1
  controller/1(u_i) -> u_i/1
  controller/2(xi_min) -> xi_i/1
  u_t,i/1(u_ti) -> Add/1
  u_d,i/1(u_di) -> Add/2
  Add/1 -> Scope1/1, Smooth Projection/1("u_mi ")
  Smooth Projection/1(u_mi) -> controller/2(u_mi), Scope2/1
  Control gain matrix/1(g_i_hat) -> controller/1(g_i_hat)

== system FO_CTDNN_P_Bia_Para_3_trigger_V1/Controller and Plant 6/Finite-time observer ==
  x_i : Inport
  u_i : Inport  Port=2
  Integrator : Integrator  InitialCondition=InitialCondition
  Multi-layer neural network : Subsystem
  Observer : MATLAB Function  TreatAsAtomicUnit=on
  x_i_tilde : Scope
  E_hat : Outport
  wires:
  x_i/1 -> Observer/2(x_i), Multi-layer neural network/2(x_i)
  u_i/1 -> Observer/3(u_i), Multi-layer neural network/3(u_i)
  Multi-layer neural network/1(E_hat) -> E_hat/1, Observer/4(E_hat)
  Observer/1(x_hat_dot) -> Integrator/1
  Integrator/1 -> Observer/1(x_i_hat)
  Observer/2(x_i_tilde) -> x_i_tilde/1, Multi-layer neural network/1(x_i_tilde)

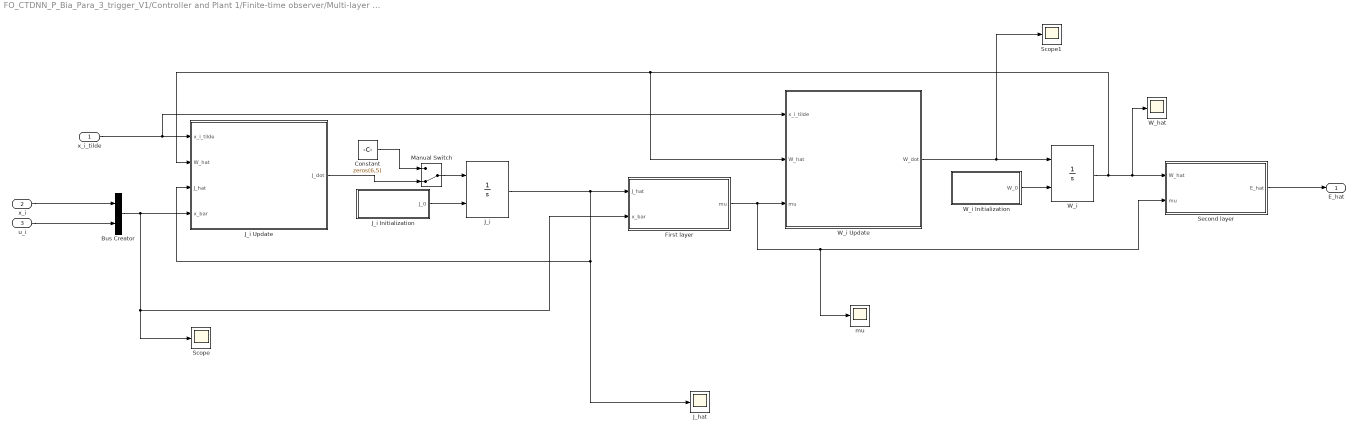
== system FO_CTDNN_P_Bia_Para_3_trigger_V1/Controller and Plant 1/Finite-time observer/Multi-layer neural network ==
  x_i_tilde : Inport
  x_i : Inport  Port=2  PortDimensions=[3,1]
  u_i : Inport  Port=3  PortDimensions=[3,1]
  Bus Creator : BusCreator  Inputs=2
  Constant : Constant  Value=zeros(6,5)
  First layer : MATLAB Function  TreatAsAtomicUnit=on
  J_hat : Scope
  J_i : Integrator  InitialConditionSource=external
  J_i Initialization : MATLAB Function  TreatAsAtomicUnit=on
  J_i Update : MATLAB Function  TreatAsAtomicUnit=on
  Manual Switch : ManualSwitch  CurrentSetting=0
  Scope : Scope
  Scope1 : Scope
  Second layer : MATLAB Function  TreatAsAtomicUnit=on
  W_hat : Scope
  W_i : Integrator  InitialConditionSource=external
  W_i Initialization : MATLAB Function  TreatAsAtomicUnit=on
  W_i Update : MATLAB Function  TreatAsAtomicUnit=on
  mu : Scope
  E_hat : Outport
  wires:
  x_i_tilde/1 -> W_i Update/1(x_i_tilde), J_i Update/1(x_i_tilde)
  W_i/1 -> W_hat/1, Second layer/1(W_hat), W_i Update/2(W_hat), J_i Update/2(W_hat)
  W_i Update/1(W_dot) -> Scope1/1, W_i/1
  W_i Initialization/1(W_0) -> W_i/2
  J_i Initialization/1(J_0) -> J_i/2
  First layer/1(mu) -> mu/1, Second layer/2(mu), W_i Update/3(mu)
  Second layer/1(E_hat) -> E_hat/1
  J_i/1 -> J_i Update/3(J_hat), J_hat/1, First layer/1(J_hat)
  Bus Creator/1 -> Scope/1, First layer/2(x_bar), J_i Update/4(x_bar)
  x_i/1 -> Bus Creator/1
  u_i/1 -> Bus Creator/2
  J_i Update/1(J_dot) -> Manual Switch/2
  Constant/1 -> Manual Switch/1
  Manual Switch/1 -> J_i/1

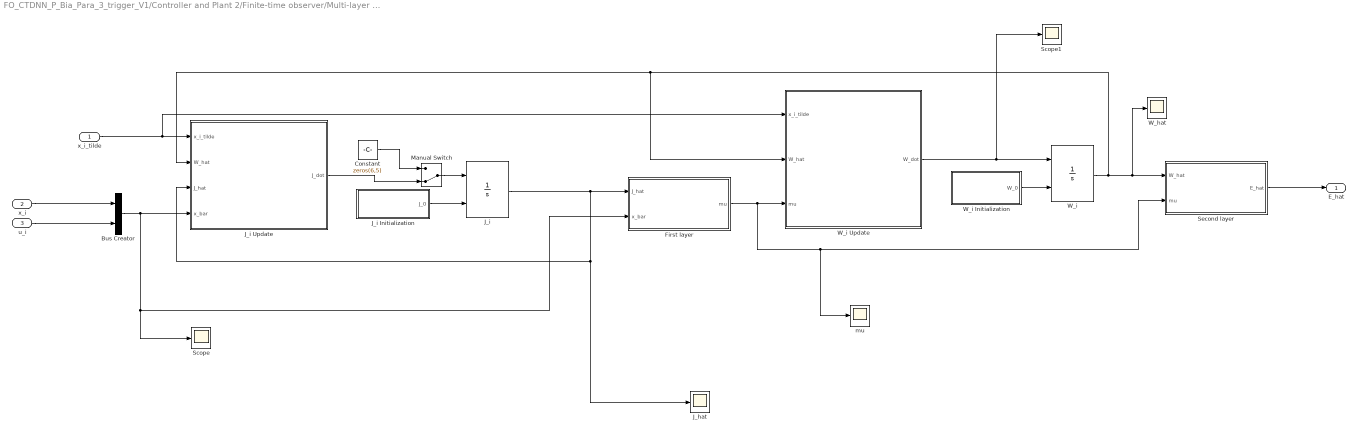
== system FO_CTDNN_P_Bia_Para_3_trigger_V1/Controller and Plant 2/Finite-time observer/Multi-layer neural network ==
  x_i_tilde : Inport
  x_i : Inport  Port=2  PortDimensions=[3,1]
  u_i : Inport  Port=3  PortDimensions=[3,1]
  Bus Creator : BusCreator  Inputs=2
  Constant : Constant  Value=zeros(6,5)
  First layer : MATLAB Function  TreatAsAtomicUnit=on
  J_hat : Scope
  J_i : Integrator  InitialConditionSource=external
  J_i Initialization : MATLAB Function  TreatAsAtomicUnit=on
  J_i Update : MATLAB Function  TreatAsAtomicUnit=on
  Manual Switch : ManualSwitch  CurrentSetting=0
  Scope : Scope
  Scope1 : Scope
  Second layer : MATLAB Function  TreatAsAtomicUnit=on
  W_hat : Scope
  W_i : Integrator  InitialConditionSource=external
  W_i Initialization : MATLAB Function  TreatAsAtomicUnit=on
  W_i Update : MATLAB Function  TreatAsAtomicUnit=on
  mu : Scope
  E_hat : Outport
  wires:
  x_i_tilde/1 -> W_i Update/1(x_i_tilde), J_i Update/1(x_i_tilde)
  W_i/1 -> W_hat/1, Second layer/1(W_hat), W_i Update/2(W_hat), J_i Update/2(W_hat)
  W_i Update/1(W_dot) -> Scope1/1, W_i/1
  W_i Initialization/1(W_0) -> W_i/2
  J_i Initialization/1(J_0) -> J_i/2
  First layer/1(mu) -> mu/1, Second layer/2(mu), W_i Update/3(mu)
  Second layer/1(E_hat) -> E_hat/1
  J_i/1 -> J_i Update/3(J_hat), J_hat/1, First layer/1(J_hat)
  Bus Creator/1 -> Scope/1, First layer/2(x_bar), J_i Update/4(x_bar)
  x_i/1 -> Bus Creator/1
  u_i/1 -> Bus Creator/2
  J_i Update/1(J_dot) -> Manual Switch/2
  Constant/1 -> Manual Switch/1
  Manual Switch/1 -> J_i/1

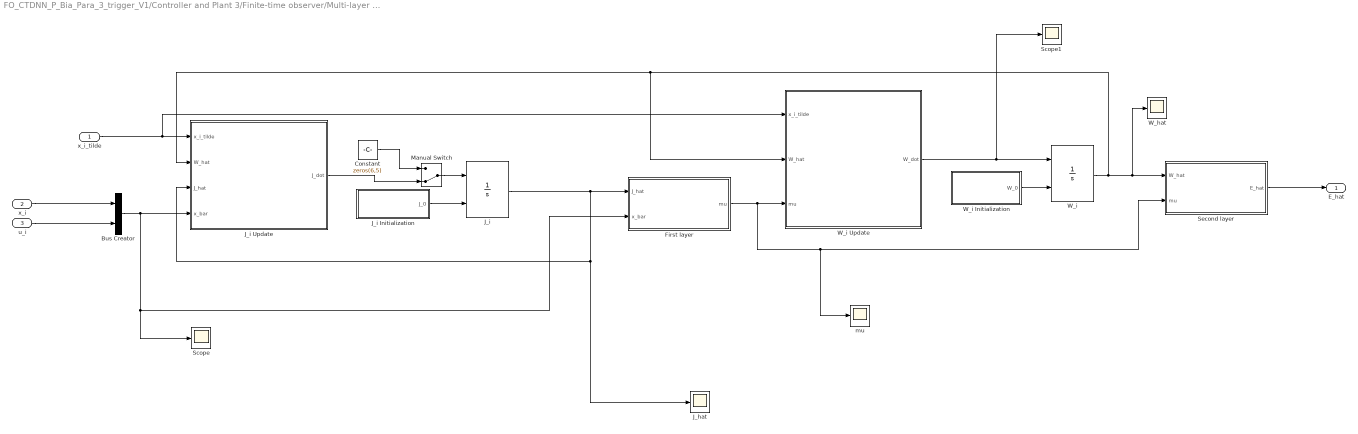
== system FO_CTDNN_P_Bia_Para_3_trigger_V1/Controller and Plant 3/Finite-time observer/Multi-layer neural network ==
  x_i_tilde : Inport
  x_i : Inport  Port=2  PortDimensions=[3,1]
  u_i : Inport  Port=3  PortDimensions=[3,1]
  Bus Creator : BusCreator  Inputs=2
  Constant : Constant  Value=zeros(6,5)
  First layer : MATLAB Function  TreatAsAtomicUnit=on
  J_hat : Scope
  J_i : Integrator  InitialConditionSource=external
  J_i Initialization : MATLAB Function  TreatAsAtomicUnit=on
  J_i Update : MATLAB Function  TreatAsAtomicUnit=on
  Manual Switch : ManualSwitch  CurrentSetting=0
  Scope : Scope
  Scope1 : Scope
  Second layer : MATLAB Function  TreatAsAtomicUnit=on
  W_hat : Scope
  W_i : Integrator  InitialConditionSource=external
  W_i Initialization : MATLAB Function  TreatAsAtomicUnit=on
  W_i Update : MATLAB Function  TreatAsAtomicUnit=on
  mu : Scope
  E_hat : Outport
  wires:
  x_i_tilde/1 -> W_i Update/1(x_i_tilde), J_i Update/1(x_i_tilde)
  W_i/1 -> W_hat/1, Second layer/1(W_hat), W_i Update/2(W_hat), J_i Update/2(W_hat)
  W_i Update/1(W_dot) -> Scope1/1, W_i/1
  W_i Initialization/1(W_0) -> W_i/2
  J_i Initialization/1(J_0) -> J_i/2
  First layer/1(mu) -> mu/1, Second layer/2(mu), W_i Update/3(mu)
  Second layer/1(E_hat) -> E_hat/1
  J_i/1 -> J_i Update/3(J_hat), J_hat/1, First layer/1(J_hat)
  Bus Creator/1 -> Scope/1, First layer/2(x_bar), J_i Update/4(x_bar)
  x_i/1 -> Bus Creator/1
  u_i/1 -> Bus Creator/2
  J_i Update/1(J_dot) -> Manual Switch/2
  Constant/1 -> Manual Switch/1
  Manual Switch/1 -> J_i/1

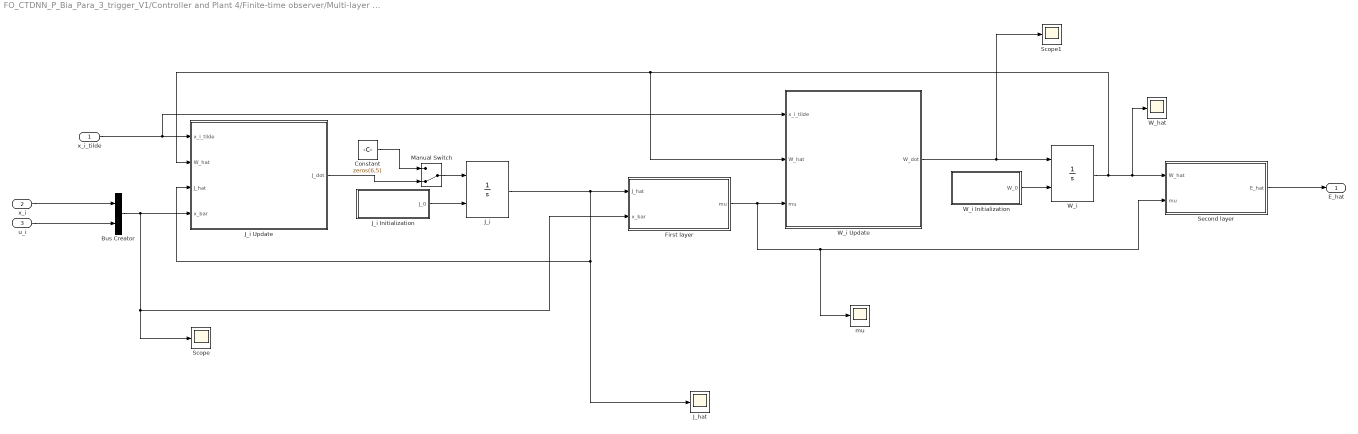
== system FO_CTDNN_P_Bia_Para_3_trigger_V1/Controller and Plant 4/Finite-time observer/Multi-layer neural network ==
  x_i_tilde : Inport
  x_i : Inport  Port=2  PortDimensions=[3,1]
  u_i : Inport  Port=3  PortDimensions=[3,1]
  Bus Creator : BusCreator  Inputs=2
  Constant : Constant  Value=zeros(6,5)
  First layer : MATLAB Function  TreatAsAtomicUnit=on
  J_hat : Scope
  J_i : Integrator  InitialConditionSource=external
  J_i Initialization : MATLAB Function  TreatAsAtomicUnit=on
  J_i Update : MATLAB Function  TreatAsAtomicUnit=on
  Manual Switch : ManualSwitch  CurrentSetting=0
  Scope : Scope
  Scope1 : Scope
  Second layer : MATLAB Function  TreatAsAtomicUnit=on
  W_hat : Scope
  W_i : Integrator  InitialConditionSource=external
  W_i Initialization : MATLAB Function  TreatAsAtomicUnit=on
  W_i Update : MATLAB Function  TreatAsAtomicUnit=on
  mu : Scope
  E_hat : Outport
  wires:
  x_i_tilde/1 -> W_i Update/1(x_i_tilde), J_i Update/1(x_i_tilde)
  W_i/1 -> W_hat/1, Second layer/1(W_hat), W_i Update/2(W_hat), J_i Update/2(W_hat)
  W_i Update/1(W_dot) -> Scope1/1, W_i/1
  W_i Initialization/1(W_0) -> W_i/2
  J_i Initialization/1(J_0) -> J_i/2
  First layer/1(mu) -> mu/1, Second layer/2(mu), W_i Update/3(mu)
  Second layer/1(E_hat) -> E_hat/1
  J_i/1 -> J_i Update/3(J_hat), J_hat/1, First layer/1(J_hat)
  Bus Creator/1 -> Scope/1, First layer/2(x_bar), J_i Update/4(x_bar)
  x_i/1 -> Bus Creator/1
  u_i/1 -> Bus Creator/2
  J_i Update/1(J_dot) -> Manual Switch/2
  Constant/1 -> Manual Switch/1
  Manual Switch/1 -> J_i/1

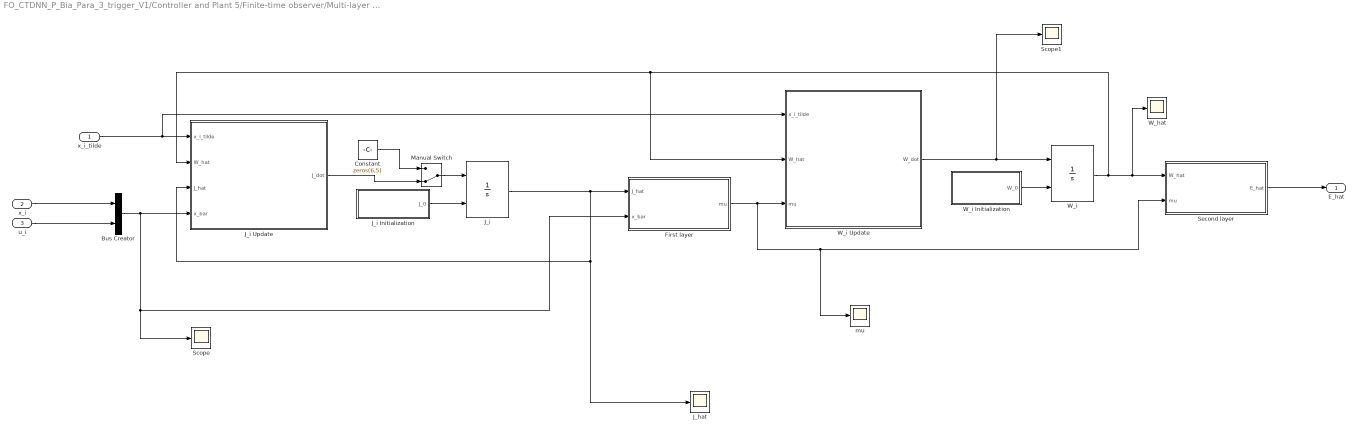
== system FO_CTDNN_P_Bia_Para_3_trigger_V1/Controller and Plant 5/Finite-time observer/Multi-layer neural network ==
  x_i_tilde : Inport
  x_i : Inport  Port=2  PortDimensions=[3,1]
  u_i : Inport  Port=3  PortDimensions=[3,1]
  Bus Creator : BusCreator  Inputs=2
  Constant : Constant  Value=zeros(6,5)
  First layer : MATLAB Function  TreatAsAtomicUnit=on
  J_hat : Scope
  J_i : Integrator  InitialConditionSource=external
  J_i Initialization : MATLAB Function  TreatAsAtomicUnit=on
  J_i Update : MATLAB Function  TreatAsAtomicUnit=on
  Manual Switch : ManualSwitch  CurrentSetting=0
  Scope : Scope
  Scope1 : Scope
  Second layer : MATLAB Function  TreatAsAtomicUnit=on
  W_hat : Scope
  W_i : Integrator  InitialConditionSource=external
  W_i Initialization : MATLAB Function  TreatAsAtomicUnit=on
  W_i Update : MATLAB Function  TreatAsAtomicUnit=on
  mu : Scope
  E_hat : Outport
  wires:
  x_i_tilde/1 -> W_i Update/1(x_i_tilde), J_i Update/1(x_i_tilde)
  W_i/1 -> W_hat/1, Second layer/1(W_hat), W_i Update/2(W_hat), J_i Update/2(W_hat)
  W_i Update/1(W_dot) -> Scope1/1, W_i/1
  W_i Initialization/1(W_0) -> W_i/2
  J_i Initialization/1(J_0) -> J_i/2
  First layer/1(mu) -> mu/1, Second layer/2(mu), W_i Update/3(mu)
  Second layer/1(E_hat) -> E_hat/1
  J_i/1 -> J_i Update/3(J_hat), J_hat/1, First layer/1(J_hat)
  Bus Creator/1 -> Scope/1, First layer/2(x_bar), J_i Update/4(x_bar)
  x_i/1 -> Bus Creator/1
  u_i/1 -> Bus Creator/2
  J_i Update/1(J_dot) -> Manual Switch/2
  Constant/1 -> Manual Switch/1
  Manual Switch/1 -> J_i/1

== system FO_CTDNN_P_Bia_Para_3_trigger_V1/Controller and Plant 6/Finite-time observer/Multi-layer neural network ==
  x_i_tilde : Inport
  x_i : Inport  Port=2  PortDimensions=[3,1]
  u_i : Inport  Port=3  PortDimensions=[3,1]
  Bus Creator : BusCreator  Inputs=2
  Constant : Constant  Value=zeros(6,5)
  First layer : MATLAB Function  TreatAsAtomicUnit=on
  J_hat : Scope
  J_i : Integrator  InitialConditionSource=external
  J_i Initialization : MATLAB Function  TreatAsAtomicUnit=on
  J_i Update : MATLAB Function  TreatAsAtomicUnit=on
  Manual Switch : ManualSwitch  CurrentSetting=0
  Scope : Scope
  Scope1 : Scope
  Second layer : MATLAB Function  TreatAsAtomicUnit=on
  W_hat : Scope
  W_i : Integrator  InitialConditionSource=external
  W_i Initialization : MATLAB Function  TreatAsAtomicUnit=on
  W_i Update : MATLAB Function  TreatAsAtomicUnit=on
  mu : Scope
  E_hat : Outport
  wires:
  x_i_tilde/1 -> W_i Update/1(x_i_tilde), J_i Update/1(x_i_tilde)
  W_i/1 -> W_hat/1, Second layer/1(W_hat), W_i Update/2(W_hat), J_i Update/2(W_hat)
  W_i Update/1(W_dot) -> Scope1/1, W_i/1
  W_i Initialization/1(W_0) -> W_i/2
  J_i Initialization/1(J_0) -> J_i/2
  First layer/1(mu) -> mu/1, Second layer/2(mu), W_i Update/3(mu)
  Second layer/1(E_hat) -> E_hat/1
  J_i/1 -> J_i Update/3(J_hat), J_hat/1, First layer/1(J_hat)
  Bus Creator/1 -> Scope/1, First layer/2(x_bar), J_i Update/4(x_bar)
  x_i/1 -> Bus Creator/1
  u_i/1 -> Bus Creator/2
  J_i Update/1(J_dot) -> Manual Switch/2
  Constant/1 -> Manual Switch/1
  Manual Switch/1 -> J_i/1

== matlab function FO_CTDNN_P_Bia_Para_3_trigger_V1/Controller and Plant 2/Controller/controller ==
  data: g_i_hat input; u_mi input; u_i output; u_ei input; xi_min output
function [u_i, xi_min]  = controller(g_i_hat, u_mi, u_ei)


%% modified saturated controller

% saturation boundary
u_m = 0.25;
dimension = 3;

u_nomi = u_mi + u_ei;
u_satu = u_nomi;


%% calculate the saturated control input first

for i = 1 : dimension
    u_satu(i) = max(min(u_satu(i), u_m), -u_m); 
end

%% judge if the reverse effect will happen

rev_flag = 0;

reu_nomi = g_i_hat * u_nomi;
reu_satu = g_i_hat * u_satu;

for i = 1 : dimension
    if reu_nomi(i) == reu_satu(i)
        continue;
    else
        rev_flag = 1;
        break;
    end
end


%% see if the algorithm should be triggered

xi = [1;1;1];

if rev_flag == 1
    % the current necessary control inputs
    u_up = u_m * ones(dimension,1) - u_mi;
    u_do = -u_m * ones(dimension,1) - u_mi;
    
    
    xi_min = 1;
    
    for i = 1:dimension
        if u_ei(i)>0
            xi(i) = u_up(i)/u_ei(i);
            xi(i) = min(xi(i), xi_min);
        elseif u_ei(i)<0
            xi(i) = u_do(i)/u_ei(i);
            xi(i) = min(xi(i), xi_min);
        else
            xi(i) = 1;
        end
    end
    
    u_i = u_mi + min(xi) * u_ei;
    
else
    u_i = u_mi + u_ei;

end


xi_min = min(xi);









end

== matlab function FO_CTDNN_P_Bia_Para_3_trigger_V1/Controller and Plant 1/Local Error Calculate ==
  data: delta_x input; e_xi output; L input
function e_xi = local_error(delta_x, L)

%% Calculate the local formation tracking error from communication

dimension = 3;
serial_num = 1;

L_i = kron(L(serial_num, :) , eye(dimension));

e_xi = L_i * delta_x;







end

== matlab function FO_CTDNN_P_Bia_Para_3_trigger_V1/Controller and Plant 2/Local Error Calculate ==
  data: delta_x input; e_xi output; L input
function e_xi = local_error(delta_x, L)

%% Calculate the local formation tracking error from communication

dimension = 3;
serial_num = 2;

L_i = kron(L(serial_num, :) , eye(dimension));

e_xi = L_i * delta_x;







end

== matlab function FO_CTDNN_P_Bia_Para_3_trigger_V1/Controller and Plant 2/Finite-time observer/Multi-layer neural network/First layer ==
  data: J_hat input; mu output; x_bar input
function mu = first_layer(J_hat, x_bar)

%% From input layer to hidden layer
% mu = tanh(J_hat * x_i)

mu = tanh(J_hat' * x_bar);

end

== matlab function FO_CTDNN_P_Bia_Para_3_trigger_V1/Controller and Plant 2/Finite-time observer/Multi-layer neural network/J_i Initialization ==
  data: J_0 output
function J_0 = J_ini()

n_1 = 5;
dimension = 3;

J_0 = rand(2*dimension,n_1);

end

== matlab function FO_CTDNN_P_Bia_Para_3_trigger_V1/Controller and Plant 2/Finite-time observer/Multi-layer neural network/J_i Update ==
  data: x_i_tilde input; J_dot output; W_hat input; J_hat input; x_bar input
function J_dot = J_update(x_i_tilde, W_hat, J_hat, x_bar)


eta_3 = 0.1;
eta_4 = 0.06;
% eta_5 = 0.1;

n_1 = 5;

alpha = tanh(J_hat' * x_bar);

% J_dot = eta_3 * sign(x_bar) * ( e_xi' * W_hat' * (eye(n_1) - diag(alpha.^2)) ) - eta_4 * norm(e_xi) * J_hat - eta_5  * J_hat; 

J_dot = eta_3 * sign(x_bar)/norm(sign(x_bar)) * ( x_i_tilde' * W_hat' * (eye(n_1) - diag(alpha.^2)) ) - eta_4 * norm(x_i_tilde) * J_hat; 

% J_dot = eta_3 * sign(x_bar) * ( e_xi' * W_hat' * (eye(n_1) - diag(alpha.^2)) ) - eta_4  * J_hat; 

end

== matlab function FO_CTDNN_P_Bia_Para_3_trigger_V1/Controller and Plant 2/Finite-time observer/Multi-layer neural network/Second layer ==
  data: W_hat input; E_hat output; mu input
function E_hat = second_layer(W_hat, mu)

%% From hidden layer to output layer
% w_hat = W_hat * mu(J_hat * x_i)


E_hat = W_hat' * mu; 

end

== matlab function FO_CTDNN_P_Bia_Para_3_trigger_V1/Controller and Plant 2/Finite-time observer/Multi-layer neural network/W_i Initialization ==
  data: W_0 output
function W_0 = W_ini()

n_1 = 5;
dimension = 3;

W_0 = 0.05*zeros(n_1,dimension);
% W_0 =randn(n, n_1);

end

== matlab function FO_CTDNN_P_Bia_Para_3_trigger_V1/Controller and Plant 1/Controller/Control gain matrix ==
  data: g_i_hat output; x_i input; g_inverse output
function [g_i_hat, g_inverse] = ctr_gain(x_i)


%% This function will estimate the system control gain matrix

Radius_esti=[0.21;0.25;0.33;0.24;0.28;0.29];

serial_num = 1;
dimension = 3; 

R_hat=Radius_esti(serial_num);

theta = x_i(dimension);

g_i_hat = [-sin(theta) -sin(pi/3 - theta) sin(pi/3 + theta);
        cos(theta) -cos(pi/3 - theta) -cos(pi/3+ theta);
        1/R_hat 1/R_hat 1/R_hat];

g_inverse = g_i_hat^(-1); 


end

== matlab function FO_CTDNN_P_Bia_Para_3_trigger_V1/Controller and Plant 2/Finite-time observer/Multi-layer neural network/W_i Update ==
  data: x_i_tilde input; W_dot output; W_hat input; mu input
function W_dot = W_update(x_i_tilde, W_hat, mu)


eta_1 = 15;
eta_2 = 0.1;
% eta_3 = 0.05;



% W_dot = eta_1 * mu * e_xi' - eta_2* norm(e_xi) * W_hat - eta_3 * W_hat; 

W_dot = eta_1 * mu * x_i_tilde' - eta_2* norm(x_i_tilde) * W_hat; 

% W_dot = eta_1 * mu * e_xi' - eta_2 * W_hat; 

end

== matlab function FO_CTDNN_P_Bia_Para_3_trigger_V1/Controller and Plant 2/Plant ==
  data: x_dot output; E_i output; x_i input; u_i input; t input
function [x_dot, E_i ] = model(x_i, u_i, t)

%% First-order plants for robots

Radius=[0.24;0.23;0.30;0.28;0.25;0.32];
Radius_esti=[0.21;0.25;0.33;0.24;0.28;0.29];

serial_num = 2;
dimension = 3; 

R = Radius(serial_num);
R_hat = Radius_esti(serial_num);

x = x_i(1);
y = x_i(2);
theta = x_i(3);

w_i =  [0.02 * cos(0.5* t+ pi/2) + 0.03 * exp( -abs(x) - 1 ) ; 0.03 * sin(0.2*t) + 0.02*tanh(y); 0.04*sin(0.1*t + theta) + 0.01 *tanh(theta)] ;
%d =  0.4* cos(0.5* t+ pi/2);


g_i = [-sin(theta) -sin(pi/3 - theta) sin(pi/3 + theta);
        cos(theta) -cos(pi/3 - theta) -cos(pi/3+ theta);
        1/R 1/R 1/R];
    
g_i_hat = [-sin(theta) -sin(pi/3 - theta) sin(pi/3 + theta);
        cos(theta) -cos(pi/3 - theta) -cos(pi/3+ theta);
        1/R_hat 1/R_hat 1/R_hat];
    
x_dot = g_i * u_i + w_i;


E_i = w_i + (g_i - g_i_hat) * u_i;




end

== matlab function FO_CTDNN_P_Bia_Para_3_trigger_V1/Self Error Calculation 2/error_calculation ==
  data: v_di output; ref input; delta_x2 output; x_i input
function [v_di, delta_x2] = error_cal(ref, x_i)

%% Basic parameters

dimension = 3;
num_agent = 6;
serial_num = 2;

x_d = ref(1+dimension*0:dimension*num_agent);
v_d = ref(1+dimension*num_agent:2*dimension*num_agent);

x_di = x_d( (serial_num - 1)*dimension+1 : serial_num*dimension );
v_di = v_d( (serial_num - 1)*dimension+1 : serial_num*dimension );



delta_x2 = x_i - x_di;


end

== matlab function FO_CTDNN_P_Bia_Para_3_trigger_V1/Controller and Plant 2/Controller/u_d,i ==
  data: g_inverse input; u_di output; w_hat input
function u_di = u_di(g_inverse, w_hat)

%% Control input for uncertainties compensation

% Smooth projection of uncertainty estimation vector
dimension = 3;

psi = 0.01;
w_m = 0.10;



for i = 1 : dimension
   if abs(w_hat(i)) <= w_m - psi
       continue;
   else
       w_hat(i) = sign(w_hat(i)) * (w_m - psi*exp( (w_m - psi - abs(w_hat(i)))/psi ));
   end 
end


u_di = - g_inverse * w_hat; 



end

== matlab function FO_CTDNN_P_Bia_Para_3_trigger_V1/Controller and Plant 2/Controller/u_e,i ==
  data: g_inverse input; u_ei output; e_xi input
function u_ei = u_ei(g_inverse, e_xi)

%% Control input for error reducing

k_p = 3;

u_ei = - k_p * g_inverse * e_xi; 



end

== matlab function FO_CTDNN_P_Bia_Para_3_trigger_V1/Controller and Plant 3/Local Error Calculate ==
  data: delta_x input; e_xi output; L input
function e_xi = local_error(delta_x, L)

%% Calculate the local formation tracking error from communication

dimension = 3;
serial_num = 3;

L_i = kron(L(serial_num, :) , eye(dimension));

e_xi = L_i * delta_x;







end

== matlab function FO_CTDNN_P_Bia_Para_3_trigger_V1/Controller and Plant 3/Finite-time observer/Multi-layer neural network/First layer ==
  data: J_hat input; mu output; x_bar input
function mu = first_layer(J_hat, x_bar)

%% From input layer to hidden layer
% mu = tanh(J_hat * x_i)

mu = tanh(J_hat' * x_bar);

end

== matlab function FO_CTDNN_P_Bia_Para_3_trigger_V1/Controller and Plant 3/Finite-time observer/Multi-layer neural network/J_i Initialization ==
  data: J_0 output
function J_0 = J_ini()

n_1 = 5;
dimension = 3;

J_0 = rand(2*dimension,n_1);

end

== matlab function FO_CTDNN_P_Bia_Para_3_trigger_V1/Controller and Plant 3/Finite-time observer/Multi-layer neural network/J_i Update ==
  data: x_i_tilde input; J_dot output; W_hat input; J_hat input; x_bar input
function J_dot = J_update(x_i_tilde, W_hat, J_hat, x_bar)


eta_3 = 0.1;
eta_4 = 0.06;
% eta_5 = 0.1;

n_1 = 5;

alpha = tanh(J_hat' * x_bar);

% J_dot = eta_3 * sign(x_bar) * ( e_xi' * W_hat' * (eye(n_1) - diag(alpha.^2)) ) - eta_4 * norm(e_xi) * J_hat - eta_5  * J_hat; 

J_dot = eta_3 * sign(x_bar)/norm(sign(x_bar)) * ( x_i_tilde' * W_hat' * (eye(n_1) - diag(alpha.^2)) ) - eta_4 * norm(x_i_tilde) * J_hat; 

% J_dot = eta_3 * sign(x_bar) * ( e_xi' * W_hat' * (eye(n_1) - diag(alpha.^2)) ) - eta_4  * J_hat; 

end

== matlab function FO_CTDNN_P_Bia_Para_3_trigger_V1/Controller and Plant 3/Finite-time observer/Multi-layer neural network/Second layer ==
  data: W_hat input; E_hat output; mu input
function E_hat = second_layer(W_hat, mu)

%% From hidden layer to output layer
% w_hat = W_hat * mu(J_hat * x_i)


E_hat = W_hat' * mu; 

end
